simulink model "CompleteModelHiL"  (R2015a)
settings: Solver=ode23  StartTime=0.0  StopTime=20000  RelTol=1e-3
StopFcn:
  | stopfun
values from neighbouring files (symbols this model uses):
  OCV_LUT = block.DialogPrm(1).Data    [AMA_sfunc.m]
undefined symbols (not defined in the file or in its folder): dec_fact, Settings
libraries: dspindex x7, Battery_Unipi x6, dsparch4 x6, simulink x3
settings Model: TunableVars=Bp2,Bp3,Cl,Cs,N,Nbits,OCV_LUT,Qr,R0,Rl,Rs,T,dec_fact,ocv,params_bp,sampletime,soc_bp,soc_init  TunableVarsStorageClass=Auto,Auto,Auto,Auto,Auto,Auto,Auto,Auto,Auto,Auto,Auto,Auto,Auto,Auto,Auto,Auto,Auto,Auto  TunableVarsTypeQualifier=,,,,,,,,,,,,,,,,,  Creator=Rocco  LastModifiedBy=pc2
settings OptimizationCC: InlineParams=on  SimCompilerOptimization=on
settings DebuggingCC: ReadBeforeWriteMsg=DisableAll  WriteAfterWriteMsg=DisableAll  WriteAfterReadMsg=DisableAll  MultiTaskDSMMsg=none
settings ModelReferenceCC: UpdateModelReferenceTargets=IfOutOfDate
settings SFSimCC: SFSimEcho=off

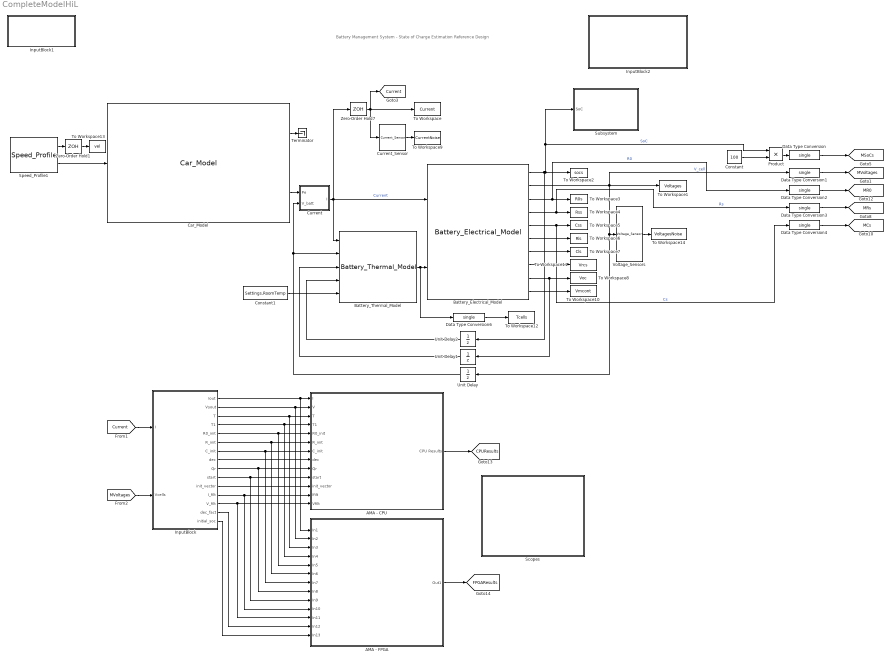
== system CompleteModelHiL ==
  note: Battery Management System - State of Charge Estimation Reference Design
  AMA - CPU : Subsystem
      mask Display: image('cpu.jpg')
  AMA - FPGA : Subsystem
      mask Display: image('max10.jpg')
  Battery_Electrical_Model : Battery_Unipi/Battery_Electrical_Model  N=Settings.N  sampletime=Settings.sampletime  Qbattery=Settings.Q  ocv=Settings.ocv  soc_bp=Settings.soc_bp  params_bp=Settings.params_bp  Ro=Settings.R0lut3d  Rs=Settings.Rslut3d  Cs=Settings.Cslut3d  Rl=Settings.Rllut3d  Cl=Settings.Cllut3d  SoC0=Settings.SoCi  Bp2=Settings.Bp2  Bp3=Settings.Bp3
      link override Cell_Model_therm: R0=Ro
  Battery_Thermal_Model : Battery_Unipi/Battery_Thermal_Model  M=Settings.N/Settings.Strings  Rthca=Settings.ThermRthca  Rthcc=Settings.ThermRthcc  Cth=Settings.ThermCap  Ta=Settings.InitTemp  sampletime=Settings.sampletime
  Car_Model : Battery_Unipi/Car_Model  M=1525  S=2.27  Cx=0.29  alphaR=0.01  roair=1.2  n_wheel=0.7  n_reg=0.5
  Constant : Constant  Value=100
  Constant1 : Constant  Value=Settings.RoomTemp
  Current : Subsystem
  Current_Sensor : Battery_Unipi/Current_Sensor  sampletime=Settings.sampletime  noisevariance=Settings.CurrVar  Nbits=Settings.CurrNbits  FS=Settings.CurrFS  Offset=Settings.CurrOff
  Data Type Conversion{,1..4,6} (6 alike) : DataTypeConversion  OutDataTypeStr=single
  InputBlock : Subsystem
  InputBlock1 : Subsystem
      mask DialogControl altera Prompt: www.altera.com
      mask Display: image('altera-logo-v3.png')
  InputBlock2 : Subsystem
      mask DialogControl altera Prompt: www.unipi.it
      mask Display: image('unipi.jpg')
  Product : Product
  Scopes : Subsystem
      mask Display: image('graph.png')
  Speed_Profile1 : Battery_Unipi/Speed_Profile  selector=Settings.profile
  Subsystem : Subsystem
      mask Display:
      | image('stop.png')
      | port_label('input', 1, 'SoC')
  Terminator : Terminator
  To Workspace : ToWorkspace  VariableName=Current  SaveFormat=Timeseries  SampleTime=-1
  To Workspace1 : ToWorkspace  VariableName=Voltages  SaveFormat=Timeseries  SampleTime=-1
  To Workspace10 : ToWorkspace  VariableName=Vmcont  SaveFormat=Timeseries  SampleTime=-1
      settings: Decimation=10
  To Workspace11 : ToWorkspace  VariableName=Vrcs  SaveFormat=Timeseries  SampleTime=-1
      settings: Decimation=10
  To Workspace12 : ToWorkspace  VariableName=Tcells  SaveFormat=Timeseries  SampleTime=-1
      settings: Decimation=10
  To Workspace13 : ToWorkspace  VariableName=vel  SaveFormat=Timeseries  SampleTime=-1
  To Workspace14 : ToWorkspace  VariableName=VoltagesNoise  SaveFormat=Timeseries  SampleTime=-1
  To Workspace2 : ToWorkspace  VariableName=socs  SaveFormat=Timeseries  SampleTime=-1
  To Workspace3 : ToWorkspace  VariableName=R0s  SaveFormat=Timeseries  SampleTime=-1
      settings: Decimation=10
  To Workspace4 : ToWorkspace  VariableName=Rss  SaveFormat=Timeseries  SampleTime=-1
      settings: Decimation=10
  To Workspace5 : ToWorkspace  VariableName=Css  SaveFormat=Timeseries  SampleTime=-1
      settings: Decimation=10
  To Workspace6 : ToWorkspace  VariableName=Rls  SaveFormat=Timeseries  SampleTime=-1
      settings: Decimation=10
  To Workspace7 : ToWorkspace  VariableName=Cls  SaveFormat=Timeseries  SampleTime=-1
      settings: Decimation=10
  To Workspace8 : ToWorkspace  VariableName=Voc  SaveFormat=Timeseries  SampleTime=-1
      settings: Decimation=10
  To Workspace9 : ToWorkspace  VariableName=CurrentNoise  SaveFormat=Timeseries  SampleTime=-1
  Unit Delay : UnitDelay  InitialCondition=4.16  SampleTime=Settings.sampletime
  Unit Delay1 : UnitDelay  InitialCondition=4.16  SampleTime=Settings.sampletime
  Unit Delay2 : UnitDelay  InitialCondition=Settings.SoCi(1)  SampleTime=Settings.sampletime
  Voltage_Sensors : Battery_Unipi/Voltage_Sensors  sampletime=Settings.sampletime  noisevariance=Settings.VoltVar  Nbits=Settings.VoltNbits  FS=Settings.VoltFS  Offset=Settings.VoltOff
  Zero-Order Hold1 : ZeroOrderHold  SampleTime=Settings.sampletime
  Zero-Order Hold7 : ZeroOrderHold  SampleTime=Settings.sampletime
  tag scope: CPUResults=global, Current=global, FPGAResults=global, MCs=global, MR0=global, MRs=global, MSoCs=global, MVoltages=global
  wires:
  Car_Model/1 -> Terminator/1
  Battery_Electrical_Model/1 -> Unit Delay2/1, Product/1, Subsystem/1(SoC), To Workspace2/1  "SoC"
  Battery_Electrical_Model/2 -> Data Type Conversion1/1, To Workspace1/1, Voltage_Sensors/1, Unit Delay/1  "V_cell"
  Battery_Electrical_Model/5 -> Data Type Conversion4/1, To Workspace5/1  "Cs"
  Battery_Electrical_Model/3 -> Data Type Conversion2/1, To Workspace3/1  "R0"
  Battery_Electrical_Model/4 -> Data Type Conversion3/1, To Workspace4/1  "Rs"
  Battery_Electrical_Model/8 -> To Workspace11/1
  Data Type Conversion6/1 -> To Workspace12/1
  Battery_Electrical_Model/6 -> To Workspace6/1
  Battery_Electrical_Model/7 -> To Workspace7/1
  Car_Model/2 -> Current/1(Pe)
  Zero-Order Hold1/1 -> To Workspace13/1
  Speed_Profile1/1 -> Zero-Order Hold1/1
  Speed_Profile1/2 -> Car_Model/1
  Zero-Order Hold7/1 -> [Current], To Workspace/1, Current_Sensor/1
  Current_Sensor/1 -> To Workspace9/1
  Current/1(I) -> Battery_Electrical_Model/1, Battery_Thermal_Model/1, Zero-Order Hold7/1  "Current"
  Battery_Electrical_Model/10 -> To Workspace10/1
  Battery_Electrical_Model/9 -> Unit Delay1/1, To Workspace8/1
  Voltage_Sensors/1 -> To Workspace14/1
  Battery_Thermal_Model/1 -> Battery_Electrical_Model/2, Data Type Conversion6/1
  Constant1/1 -> Battery_Thermal_Model/5
  Unit Delay/1 -> Battery_Thermal_Model/2, Current/2(V_batt)
  Unit Delay1/1 -> Battery_Thermal_Model/3
  Unit Delay2/1 -> Battery_Thermal_Model/4
  InputBlock/1(Iout) -> AMA - FPGA/1(In1), AMA - CPU/1(I)
  InputBlock/2(Vsout) -> AMA - FPGA/2(In2), AMA - CPU/2(V)
  InputBlock/3(T) -> AMA - FPGA/3(In3), AMA - CPU/3(T)
  InputBlock/4(T1) -> AMA - FPGA/4(In4), AMA - CPU/4(T1)
  InputBlock/6(R_init) -> AMA - FPGA/6(In6), AMA - CPU/6(R_init)
  [Current] -> InputBlock/1(I)
  [MVoltages] -> InputBlock/2(Vcells)
  InputBlock/5("R0_init ") -> AMA - FPGA/5(In5), AMA - CPU/5(R0_init)
  InputBlock/7(C_init) -> AMA - FPGA/7(In7), AMA - CPU/7(C_init)
  InputBlock/8(dec) -> AMA - CPU/8(dec)
  InputBlock/9(Qr) -> AMA - FPGA/8(In8), AMA - CPU/9(Qr)
  InputBlock/10("start ") -> AMA - FPGA/9(In9), AMA - CPU/10(start)
  InputBlock/11(init_vector) -> AMA - CPU/11(init_vector)
  InputBlock/12(I_filt) -> AMA - FPGA/10(In10), AMA - CPU/12(Ifilt)
  InputBlock/13(V_filt) -> AMA - FPGA/11(In11), AMA - CPU/13(Vfilt)
  InputBlock/14(dec_fact) -> AMA - FPGA/12(In12)
  InputBlock/15(initial_soc) -> AMA - FPGA/13(In13)
  AMA - CPU/1(CPU Results) -> [CPUResults]
  AMA - FPGA/1(Out1) -> [FPGAResults]
  Data Type Conversion/1 -> [MSoCs]
  Data Type Conversion1/1 -> [MVoltages]
  Data Type Conversion4/1 -> [MCs]
  Data Type Conversion3/1 -> [MRs]
  Data Type Conversion2/1 -> [MR0]
  Product/1 -> Data Type Conversion/1
  Constant/1 -> Product/2

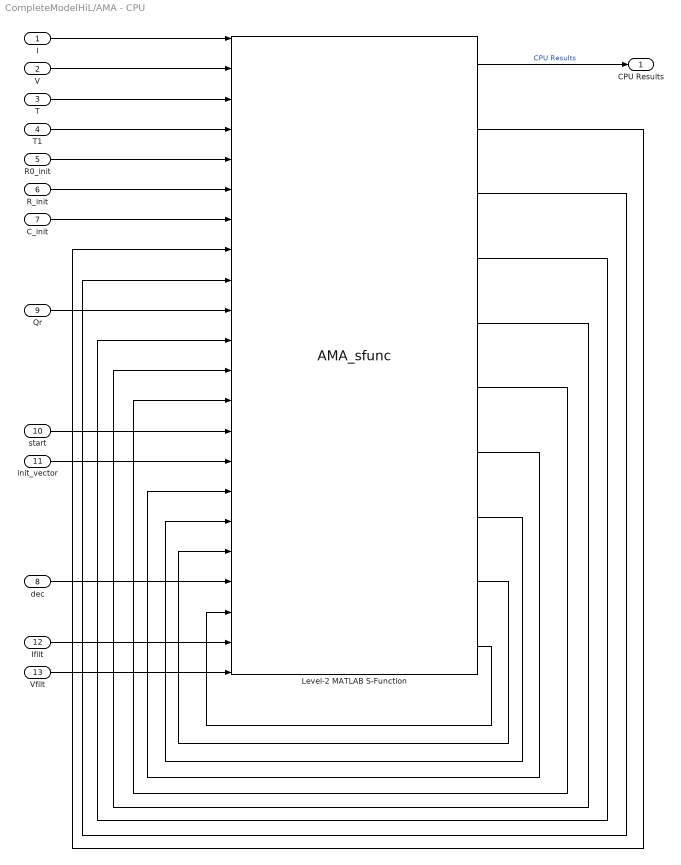
== system CompleteModelHiL/AMA - CPU ==
  I : Inport
  V : Inport  Port=2
  T : Inport  Port=3
  T1 : Inport  Port=4
  R0_init : Inport  Port=5
  R_init : Inport  Port=6
  C_init : Inport  Port=7
  dec : Inport  Port=8
  Qr : Inport  Port=9
  start : Inport  Port=10
  init_vector : Inport  Port=11
  Ifilt : Inport  Port=12
  Vfilt : Inport  Port=13
  Level-2 MATLAB S-Function : M-S-Function  FunctionName=AMA_sfunc  Parameters=single(OCV_LUT)
  CPU Results : Outport
  wires:
  R_init/1 -> Level-2 MATLAB S-Function/6
  V/1 -> Level-2 MATLAB S-Function/2
  dec/1 -> Level-2 MATLAB S-Function/19
  C_init/1 -> Level-2 MATLAB S-Function/7
  I/1 -> Level-2 MATLAB S-Function/1
  T/1 -> Level-2 MATLAB S-Function/3
  T1/1 -> Level-2 MATLAB S-Function/4
  Level-2 MATLAB S-Function/6 -> Level-2 MATLAB S-Function/13
  Level-2 MATLAB S-Function/5 -> Level-2 MATLAB S-Function/12
  Level-2 MATLAB S-Function/2 -> Level-2 MATLAB S-Function/8
  Level-2 MATLAB S-Function/1 -> CPU Results/1  "CPU Results"
  Level-2 MATLAB S-Function/4 -> Level-2 MATLAB S-Function/11
  Level-2 MATLAB S-Function/3 -> Level-2 MATLAB S-Function/9
  Level-2 MATLAB S-Function/9 -> Level-2 MATLAB S-Function/18
  Level-2 MATLAB S-Function/8 -> Level-2 MATLAB S-Function/17
  Level-2 MATLAB S-Function/7 -> Level-2 MATLAB S-Function/16
  Level-2 MATLAB S-Function/10 -> Level-2 MATLAB S-Function/20
  Ifilt/1 -> Level-2 MATLAB S-Function/21
  Vfilt/1 -> Level-2 MATLAB S-Function/22
  R0_init/1 -> Level-2 MATLAB S-Function/5
  Qr/1 -> Level-2 MATLAB S-Function/10
  start/1 -> Level-2 MATLAB S-Function/14
  init_vector/1 -> Level-2 MATLAB S-Function/15

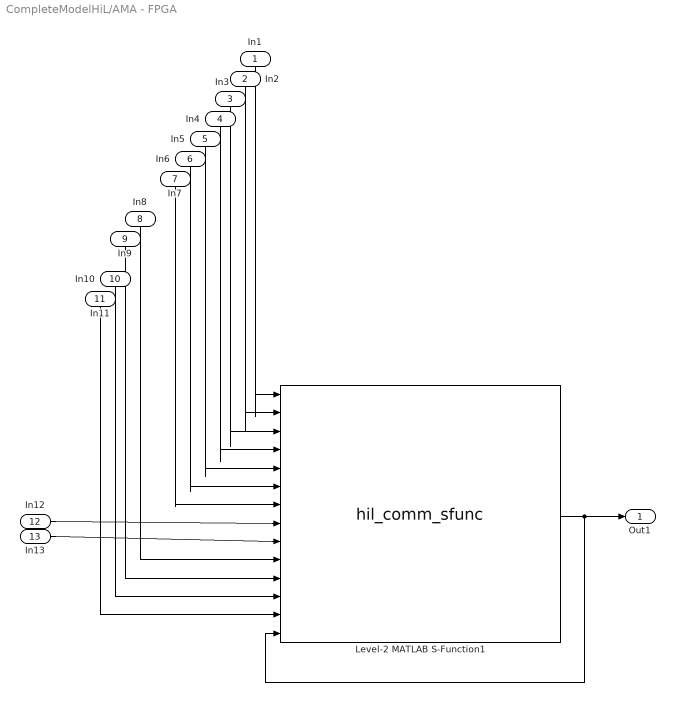
== system CompleteModelHiL/AMA - FPGA ==
  In1 : Inport
  In2 : Inport  Port=2
  In3 : Inport  Port=3
  In4 : Inport  Port=4
  In5 : Inport  Port=5
  In6 : Inport  Port=6
  In7 : Inport  Port=7
  In8 : Inport  Port=8
  In9 : Inport  Port=9
  In10 : Inport  Port=10
  In11 : Inport  Port=11
  In12 : Inport  Port=12
  In13 : Inport  Port=13
  Level-2 MATLAB S-Function1 : M-S-Function  FunctionName=hil_comm_sfunc
  Out1 : Outport
  wires:
  Level-2 MATLAB S-Function1/1 -> Out1/1, Level-2 MATLAB S-Function1/14
  In12/1 -> Level-2 MATLAB S-Function1/8
  In13/1 -> Level-2 MATLAB S-Function1/9
  In3/1 -> Level-2 MATLAB S-Function1/3
  In5/1 -> Level-2 MATLAB S-Function1/5
  In9/1 -> Level-2 MATLAB S-Function1/11
  In6/1 -> Level-2 MATLAB S-Function1/6
  In4/1 -> Level-2 MATLAB S-Function1/4
  In10/1 -> Level-2 MATLAB S-Function1/12
  In11/1 -> Level-2 MATLAB S-Function1/13
  In1/1 -> Level-2 MATLAB S-Function1/1
  In2/1 -> Level-2 MATLAB S-Function1/2
  In7/1 -> Level-2 MATLAB S-Function1/7
  In8/1 -> Level-2 MATLAB S-Function1/10

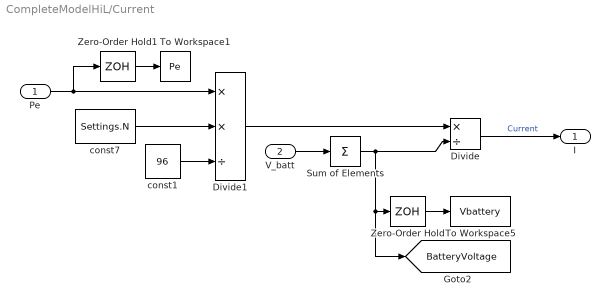
== system CompleteModelHiL/Current ==
  Pe : Inport
  V_batt : Inport  Port=2
  Divide : Product  Inputs=*/
  Divide1 : Product  Inputs=**/
  Sum of Elements : Sum  Inputs=+
  To Workspace1 : ToWorkspace  VariableName=Pe  SaveFormat=Timeseries  SampleTime=-1
      settings: Decimation=10
  To Workspace5 : ToWorkspace  VariableName=Vbattery  SaveFormat=Timeseries  SampleTime=-1
      settings: Decimation=10
  Zero-Order Hold : ZeroOrderHold  SampleTime=Settings.sampletime
  Zero-Order Hold1 : ZeroOrderHold  SampleTime=Settings.sampletime
  const1 : Constant  Value=96  OutDataTypeStr=single  SampleTime=Inf
  const7 : Constant  Value=Settings.N  OutDataTypeStr=single  SampleTime=Inf
  I : Outport
  tag scope: BatteryVoltage=global
  wires:
  Divide1/1 -> Divide/1
  const1/1 -> Divide1/3
  V_batt/1 -> Sum of Elements/1
  Sum of Elements/1 -> Divide/2, [BatteryVoltage], Zero-Order Hold/1
  const7/1 -> Divide1/2
  Pe/1 -> Zero-Order Hold1/1, Divide1/1
  Divide/1 -> I/1  "Current"
  Zero-Order Hold/1 -> To Workspace5/1
  Zero-Order Hold1/1 -> To Workspace1/1

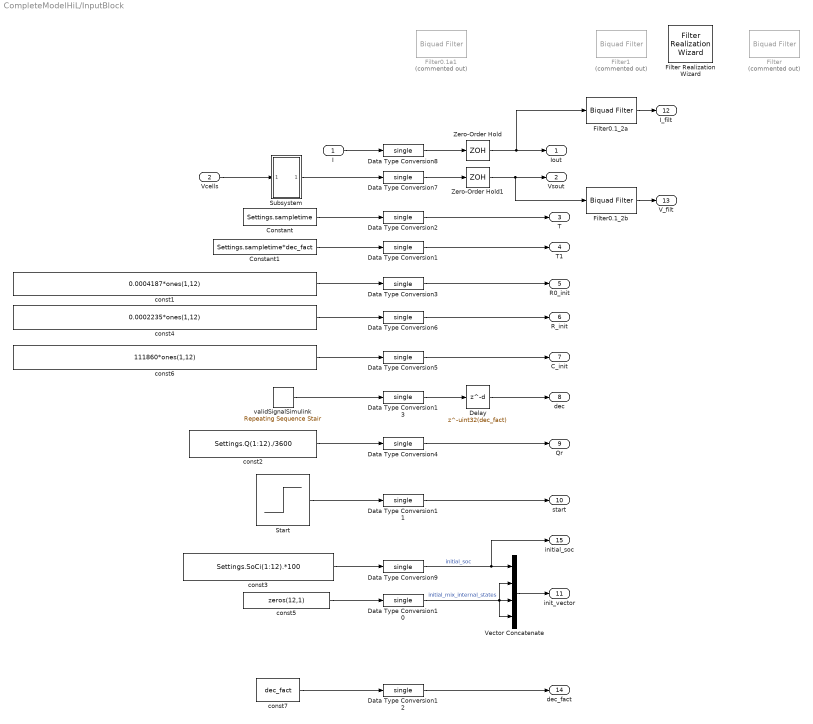
== system CompleteModelHiL/InputBlock ==
  I : Inport
  Vcells : Inport  Port=2
  Constant : Constant  Value=Settings.sampletime  SampleTime=Inf
  Constant1 : Constant  Value=Settings.sampletime*dec_fact  SampleTime=Inf
  Data Type Conversion{1..13} (13 alike) : DataTypeConversion  OutDataTypeStr=single
  Delay : Delay  DelayLength=uint32(dec_fact)  InitialCondition=0  SampleTime=Settings.sampletime
  Filter : dsparch4/Biquad Filter  Tag=BlockMethodSubSystem  Commented=on  IIRFiltStruct=Direct form II  CoeffSource=Specify via dialog  BiQuadCoeffs=[1 -0.37937622398720183 1 1 -1.977761162516769 0.98296154355766985;1 0.057146936114785295 1 1 -1.9491207799698551 0.95293889396365183;1 1.0984661154472131 1 1 -1.9304579283177468 0.93262490079303551;1 1 0 1 -0.96200755126336446 0]  a0Flag=Warning  IC=0  ICnum=0  ICden=0  InputProcessing=Columns as channels (frame based)  denAccumFracLength=30  denProdOutputFracLength=30  secondMemoryFracLength=15  roundingMode=Floor  overflowMode=off  ScaleValues=[0.0019772281687409085;0.0018560239556868123;0.00069936942814560613;0.030829285642533205;1]  optimizeScaleValues=on  ScaleValueMode=Specify via input port (g)  scaleValueFracLength=14  FilterSource=Specify via dialog  FilterObject=Hm_biquad
  Filter Realization Wizard : dsparch4/Filter Realization Wizard
  Filter0.1_2a : dsparch4/Biquad Filter  Tag=BlockMethodSubSystem  IIRFiltStruct=Direct form II  CoeffSource=Specify via dialog  BiQuadCoeffs=[1 1 0 1 -0.99790778897276833 0]  a0Flag=Warning  IC=0  ICnum=0  ICden=0  denAccumFracLength=30  denProdOutputFracLength=30  secondMemoryFracLength=15  roundingMode=Floor  overflowMode=off  ScaleValues=[0.001046105513615904;1]  optimizeScaleValues=on  ScaleValueMode=Specify via input port (g)  scaleValueFracLength=14  FilterSource=Specify via dialog  FilterObject=Hm_biquad
  "Filter0.1_2b " : dsparch4/Biquad Filter  Tag=BlockMethodSubSystem  IIRFiltStruct=Direct form II  CoeffSource=Specify via dialog  BiQuadCoeffs=[1 1 0 1 -0.99790778897276833 0]  a0Flag=Warning  IC=0  ICnum=0  ICden=0  denAccumFracLength=30  denProdOutputFracLength=30  secondMemoryFracLength=15  roundingMode=Floor  overflowMode=off  ScaleValues=[0.001046105513615904;1]  optimizeScaleValues=on  ScaleValueMode=Specify via input port (g)  scaleValueFracLength=14  FilterSource=Specify via dialog  FilterObject=Hm_biquad
  Filter0.1a1 : dsparch4/Biquad Filter  Tag=BlockMethodSubSystem  Commented=on  IIRFiltStruct=Direct form II  CoeffSource=Specify via dialog  BiQuadCoeffs=[1 -1.974309254937566 1 1 -1.9842757746773929 0.98623529999021375;1 -1.9604651825243573 1 1 -1.9593020720948617 0.96094998178536073;1 -1.8754678756966003 1 1 -1.9410248958076679 0.94228507783406268;1 1 0 1 -0.96707816729661034 0]  a0Flag=Warning  IC=0  ICnum=0  ICden=0  denAccumFracLength=30  denProdOutputFracLength=30  secondMemoryFracLength=15  roundingMode=Floor  overflowMode=off  ScaleValues=[0.081260776057318698;0.041682491427062374;0.010119332930712415;0.015450666585834652;1]  optimizeScaleValues=on  ScaleValueMode=Specify via input port (g)  scaleValueFracLength=14  FilterSource=Specify via dialog  FilterObject=Hm_biquad
  Filter1 : dsparch4/Biquad Filter  Tag=BlockMethodSubSystem  Commented=on  IIRFiltStruct=Direct form II  CoeffSource=Specify via dialog  BiQuadCoeffs=[1 -1.7798091534496587 1 1 -1.9420457145983858 0.95939749742566494;1 -1.6698605330873366 1 1 -1.8732930828757175 0.8875398987247719;1 -1.1017802038646665 1 1 -1.8258831781403617 0.83659394313774715;1 1 0 1 -0.90432244987210342 0]  a0Flag=Warning  IC=0  ICnum=0  ICden=0  denAccumFracLength=30  denProdOutputFracLength=30  secondMemoryFracLength=15  roundingMode=Floor  overflowMode=off  ScaleValues=[0.083955978843298612;0.043153931222719252;0.011924436583862363;0.044902783514339607;1]  optimizeScaleValues=on  ScaleValueMode=Specify via input port (g)  scaleValueFracLength=14  FilterSource=Specify via dialog  FilterObject=Hm_biquad
  Start : Step  Time=Settings.sampletime  Before=1  After=0  SampleTime=Settings.sampletime
      mask Display: image('engine_start.jpg')
  Subsystem : Subsystem
  Vector Concatenate : Concatenate  NumInputs=4  Mode=Multidimensional array  ConcatenateDimension=2
  Zero-Order Hold : ZeroOrderHold  SampleTime=Settings.sampletime
  Zero-Order Hold1 : ZeroOrderHold  SampleTime=Settings.sampletime
  const1 : Constant  Value=0.0004187*ones(1,12)  OutDataTypeStr=single  SampleTime=Inf
  const2 : Constant  Value=Settings.Q(1:12)./3600  OutDataTypeStr=single  SampleTime=Inf
  const3 : Constant  Value=Settings.SoCi(1:12).*100  OutDataTypeStr=single  SampleTime=Inf
  const4 : Constant  Value=0.0002235*ones(1,12)  OutDataTypeStr=single  SampleTime=Inf
  const5 : Constant  Value=zeros(12,1)  OutDataTypeStr=single  SampleTime=Inf
  const6 : Constant  Value=111860*ones(1,12)  OutDataTypeStr=single  SampleTime=Inf
  const7 : Constant  Value=dec_fact  OutDataTypeStr=single  SampleTime=Inf
  validSignalSimulink : simulink/Sources/Repeating Sequence Stair  OutValues=[1 zeros(1,dec_fact-1)]  tsamp=Settings.sampletime  OutMin=[]  OutMax=[]  OutDataTypeStr=fixdt('boolean')  OutputDataTypeScalingMode=Specify via dialog  OutDataType=fixdt('boolean')  ConRadixGroup=Best Precision: Vector-wise  OutScaling=[]
  Iout : Outport
  Vsout : Outport  Port=2
  T : Outport  Port=3
  T1 : Outport  Port=4
  "R0_init " : Outport  Port=5
  R_init : Outport  Port=6
  C_init : Outport  Port=7
  dec : Outport  Port=8
  Qr : Outport  Port=9
  "start " : Outport  Port=10
  init_vector : Outport  Port=11
  I_filt : Outport  Port=12
  V_filt : Outport  Port=13
  dec_fact : Outport  Port=14
  initial_soc : Outport  Port=15
  wires:
  const4/1 -> Data Type Conversion6/1
  Data Type Conversion1/1 -> T1/1
  Constant1/1 -> Data Type Conversion1/1
  Data Type Conversion2/1 -> T/1
  Constant/1 -> Data Type Conversion2/1
  Data Type Conversion8/1 -> Zero-Order Hold/1
  Data Type Conversion6/1 -> R_init/1
  I/1 -> Data Type Conversion8/1
  const1/1 -> Data Type Conversion3/1
  Data Type Conversion3/1 -> "R0_init "/1
  const6/1 -> Data Type Conversion5/1
  Data Type Conversion5/1 -> C_init/1
  validSignalSimulink/1 -> Data Type Conversion13/1
  Data Type Conversion13/1 -> Delay/1
  Delay/1 -> dec/1
  const2/1 -> Data Type Conversion4/1
  Data Type Conversion4/1 -> Qr/1
  Start/1 -> Data Type Conversion11/1
  Data Type Conversion11/1 -> "start "/1
  const3/1 -> Data Type Conversion9/1
  const5/1 -> Data Type Conversion10/1
  Data Type Conversion10/1 -> Vector Concatenate/2, Vector Concatenate/4, Vector Concatenate/3  "initial_mix_internal_states"
  Data Type Conversion9/1 -> initial_soc/1, Vector Concatenate/1  "initial_soc"
  Vector Concatenate/1 -> init_vector/1
  Zero-Order Hold/1 -> Filter0.1_2a/1, Iout/1
  Filter0.1_2a/1 -> I_filt/1
  "Filter0.1_2b "/1 -> V_filt/1
  const7/1 -> Data Type Conversion12/1
  Data Type Conversion12/1 -> dec_fact/1
  Vcells/1 -> Subsystem/1(In2)
  Subsystem/1(Out2) -> Data Type Conversion7/1
  Data Type Conversion7/1 -> Zero-Order Hold1/1
  Zero-Order Hold1/1 -> "Filter0.1_2b "/1, Vsout/1

== system CompleteModelHiL/InputBlock1 ==

== system CompleteModelHiL/InputBlock2 ==

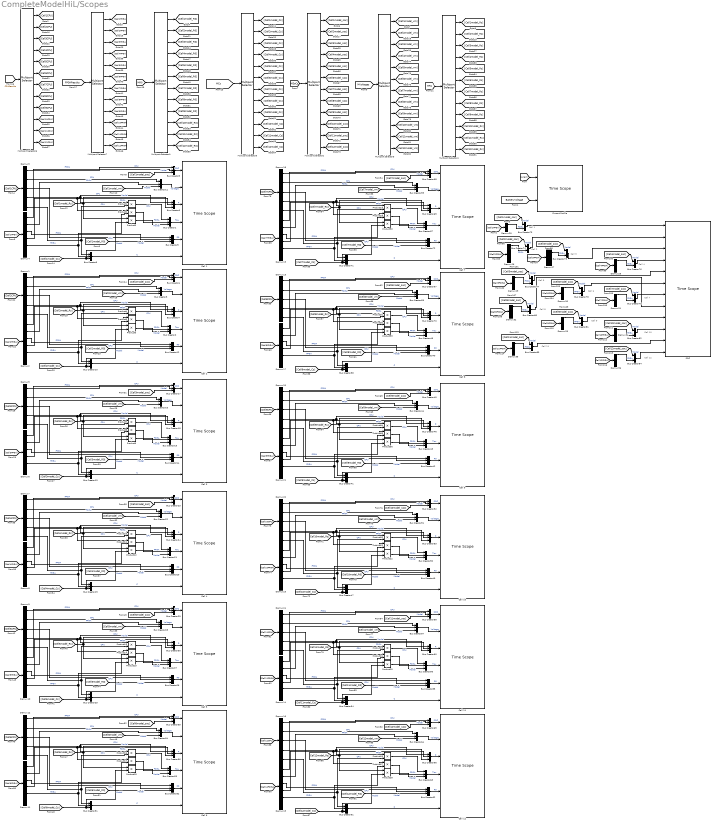
== system CompleteModelHiL/Scopes ==
  note: Cell 1
  note: Cell 2
  note: Cell 3
  note: Cell 4
  note: Cell 5
  note: Cell 6
  note: Cell 7
  note: Cell 8
  note: Cell 9
  note: Cell 10
  note: Cell 11
  note: Cell 12
  Bus Creator{1..72} (72 alike) : BusCreator  Inputs=3
  Bus Creator{73..84} (12 alike) : BusCreator  Inputs=2
  Cell {1..12} (12 alike) : TimeScope  DefaultConfigurationName=spbscopes.TimeScopeBlockCfg  NumInputPorts=6
  Current Profile : TimeScope  DefaultConfigurationName=spbscopes.TimeScopeBlockCfg  NumInputPorts=2
  Demux{1,3,5,7,9,12..13,16,18,20,22,24} (12 alike) : Demux  Outputs=5
  Demux{2,4,6,8,10..11,14..15,17,19,21,23,25..36} (24 alike) : Demux  Outputs=6
  Multiport Selector{1..7} (7 alike) : dspindex/Multiport Selector  rowsOrCols=Rows  idxCellArray={1,2,3,4,5,6,7,8,9,10,11,12 }  idxErrMode=Clip Index
  Product{1..36} (36 alike) : Product
  SOC : TimeScope  DefaultConfigurationName=spbscopes.TimeScopeBlockCfg  NumInputPorts=12
  wires:
  [Cell1model_Cs] -> Product3/2, Bus Creator8/3  "Model"
  [MSoCs] -> Multiport Selector2/1
  [Cell1model_R0] -> Bus Creator9/3  "Model"
  Multiport Selector3/1 -> [Cell1model_vm]
  Multiport Selector5/1 -> [Cell1model_Cs]
  Bus Creator11/1 -> Cell 1/2  "Voltage"
  Demux3/4 -> Bus Creator6/1, Product1/1  "CPU"
  Demux4/1 -> Bus Creator5/2  "FPGA"
  Bus Creator6/1 -> Cell 1/3  "R"
  Demux3/1 -> Bus Creator5/1  "CPU"
  Demux4/2 -> Bus Creator11/2  "FPGA"
  Multiport Selector2/1 -> [Cell1model_soc]
  Bus Creator5/1 -> Cell 1/1  "SOC"
  Product1/1 -> Bus Creator1/1  "CPU"
  Bus Creator8/1 -> Cell 1/6  "C"
  Bus Creator9/1 -> Cell 1/5  "R0"
  Demux3/2 -> Bus Creator11/1  "CPU"
  Multiport Selector5/11 -> [Cell11model_Cs]
  Multiport Selector2/4 -> [Cell4model_soc]
  Multiport Selector2/5 -> [Cell5model_soc]
  Multiport Selector3/8 -> [Cell8model_vm]
  Multiport Selector2/6 -> [Cell6model_soc]
  Product6/1 -> Bus Creator2/3  "Model"
  [Cell2CPU] -> Demux1/1
  Bus Creator4/1 -> Cell 2/1  "SOC"
  Multiport Selector1/3 -> [Cell3model_R0]
  Demux1/4 -> Product4/1, Bus Creator7/1  "CPU"
  Bus Creator3/1 -> Cell 2/2  "Voltage"
  Product4/1 -> Bus Creator2/1  "CPU"
  Multiport Selector3/3 -> [Cell3model_vm]
  Multiport Selector3/9 -> [Cell9model_vm]
  Demux1/2 -> Bus Creator3/1  "CPU"
  [CPUResults] -> Multiport Selector6/1
  [Cell2model_soc] -> Bus Creator4/3  "Model"
  Bus Creator7/1 -> Cell 2/3  "R"
  Demux2/4 -> Bus Creator7/2, Product5/1  "FPGA"
  Demux2/3 -> Bus Creator12/2  "FPGA"
  Demux2/1 -> Bus Creator4/2  "FPGA"
  Demux1/3 -> Bus Creator12/1  "CPU"
  Demux1/5 -> Bus Creator10/1, Product4/2  "CPU"
  [Cell2model_Cs] -> Bus Creator10/3, Product6/2  "Model"
  [Cell2model_vm] -> Bus Creator3/3  "Model"
  Multiport Selector3/6 -> [Cell6model_vm]
  Multiport Selector3/4 -> [Cell4model_vm]
  [Cell2model_Rs] -> Bus Creator7/3, Product6/1  "Model"
  Demux2/5 -> Bus Creator10/2, Product5/2  "FPGA"
  Bus Creator10/1 -> Cell 2/6  "C"
  Product5/1 -> Bus Creator2/2  "FPGA"
  [Cell2model_R0] -> Bus Creator12/3  "Model"
  Multiport Selector7/3 -> [Cell3FPGA]
  Bus Creator2/1 -> Cell 2/4  "Tau"
  Multiport Selector2/3 -> [Cell3model_soc]
  Demux2/2 -> Bus Creator3/2  "FPGA"
  Bus Creator12/1 -> Cell 2/5  "R0"
  Multiport Selector1/7 -> [Cell7model_R0]
  [Cell2FPGA] -> Demux2/1
  Demux1/1 -> Bus Creator4/1  "CPU"
  Multiport Selector6/5 -> [Cell5CPU]
  Multiport Selector2/10 -> [Cell10model_soc]
  Multiport Selector1/11 -> [Cell11model_R0]
  Multiport Selector7/4 -> [Cell4FPGA]
  Multiport Selector3/5 -> [Cell5model_vm]
  Multiport Selector7/9 -> [Cell9FPGA]
  Multiport Selector2/11 -> [Cell11model_soc]
  Multiport Selector1/5 -> [Cell5model_R0]
  Multiport Selector6/2 -> [Cell2CPU]
  Multiport Selector4/5 -> [Cell5model_Rs]
  Multiport Selector7/5 -> [Cell5FPGA]
  Multiport Selector5/7 -> [Cell7model_Cs]
  Multiport Selector4/12 -> [Cell12model_Rs]
  Multiport Selector4/8 -> [Cell8model_Rs]
  Multiport Selector1/4 -> [Cell4model_R0]
  Multiport Selector4/3 -> [Cell3model_Rs]
  Multiport Selector3/2 -> [Cell2model_vm]
  Multiport Selector4/4 -> [Cell4model_Rs]
  Multiport Selector4/9 -> [Cell9model_Rs]
  Multiport Selector2/12 -> [Cell12model_soc]
  Multiport Selector7/10 -> [Cell10FPGA]
  Multiport Selector1/10 -> [Cell10model_R0]
  Multiport Selector2/2 -> [Cell2model_soc]
  Multiport Selector5/9 -> [Cell9model_Cs]
  Multiport Selector2/7 -> [Cell7model_soc]
  Multiport Selector5/2 -> [Cell2model_Cs]
  Multiport Selector3/12 -> [Cell12model_vm]
  Multiport Selector5/3 -> [Cell3model_Cs]
  Multiport Selector7/2 -> [Cell2FPGA]
  Multiport Selector5/5 -> [Cell5model_Cs]
  Multiport Selector1/12 -> [Cell12model_R0]
  Multiport Selector1/6 -> [Cell6model_R0]
  Multiport Selector1/8 -> [Cell8model_R0]
  Multiport Selector6/4 -> [Cell4CPU]
  Multiport Selector7/1 -> [Cell1FPGA]
  Demux4/3 -> Bus Creator9/2  "FPGA"
  Demux3/3 -> Bus Creator9/1  "CPU"
  Demux3/5 -> Product1/2, Bus Creator8/1  "CPU"
  [MCs] -> Multiport Selector5/1
  [Cell1CPU] -> Demux3/1
  [MRs] -> Multiport Selector4/1
  [Cell1FPGA] -> Demux4/1
  Demux4/5 -> Product2/2, Bus Creator8/2  "FPGA"
  Multiport Selector4/1 -> [Cell1model_Rs]
  [Cell1model_Rs] -> Product3/1, Bus Creator6/3  "Model"
  [Cell1model_vm] -> Bus Creator11/3  "Model"
  [MVoltages] -> Multiport Selector3/1
  Demux4/4 -> Product2/1, Bus Creator6/2  "FPGA"
  Multiport Selector6/1 -> [Cell1CPU]
  [MR0] -> Multiport Selector1/1
  [Cell1model_soc] -> Bus Creator5/3  "Model"
  Multiport Selector1/1 -> [Cell1model_R0]
  Demux5/5 -> Product7/2, Bus Creator13/1  "CPU"
  Demux5/4 -> Bus Creator18/1, Product7/1  "CPU"
  [Cell5FPGA] -> Demux10/1
  Product7/1 -> Bus Creator15/1  "CPU"
  Demux7/1 -> Bus Creator23/1  "CPU"
  Demux6/2 -> Bus Creator16/2  "FPGA"
  Demux6/5 -> Product8/2, Bus Creator13/2  "FPGA"
  Bus Creator28/1 -> Cell 5/2  "Voltage"
  Multiport Selector6/10 -> [Cell10CPU]
  Bus Creator13/1 -> Cell 3/6  "C"
  [Cell3model_vm] -> Bus Creator16/3  "Model"
  Demux9/5 -> Product13/2, Bus Creator25/1  "CPU"
  Demux10/4 -> Product14/1, Bus Creator30/2  "FPGA"
  Multiport Selector3/7 -> [Cell7model_vm]
  Demux7/2 -> Bus Creator22/1  "CPU"
  Multiport Selector5/10 -> [Cell10model_Cs]
  Multiport Selector7/11 -> [Cell11FPGA]
  Bus Creator26/1 -> Cell 5/5  "R0"
  Bus Creator15/1 -> Cell 3/4  "Tau"
  Multiport Selector1/9 -> [Cell9model_R0]
  Demux8/3 -> Bus Creator20/2  "FPGA"
  Demux10/3 -> Bus Creator26/2  "FPGA"
  Product15/1 -> Bus Creator27/3  "Model"
  Product10/1 -> Bus Creator21/1  "CPU"
  Product11/1 -> Bus Creator21/2  "FPGA"
  Product13/1 -> Bus Creator27/1  "CPU"
  Demux6/4 -> Product8/1, Bus Creator18/2  "FPGA"
  Multiport Selector4/10 -> [Cell10model_Rs]
  Demux8/4 -> Bus Creator24/2, Product11/1  "FPGA"
  Multiport Selector6/7 -> [Cell7CPU]
  [Cell5model_Cs] -> Product15/2, Bus Creator25/3  "Model"
  Demux8/1 -> Bus Creator23/2  "FPGA"
  [Cell5model_Rs] -> Product15/1, Bus Creator30/3  "Model"
  Demux10/1 -> Bus Creator29/2  "FPGA"
  Multiport Selector6/3 -> [Cell3CPU]
  [Cell3CPU] -> Demux5/1
  Multiport Selector4/2 -> [Cell2model_Rs]
  Multiport Selector3/10 -> [Cell10model_vm]
  Multiport Selector5/6 -> [Cell6model_Cs]
  [Cell5model_vm] -> Bus Creator28/3  "Model"
  Bus Creator27/1 -> Cell 5/4  "Tau"
  Product12/1 -> Bus Creator21/3  "Model"
  Bus Creator24/1 -> Cell 4/3  "R"
  Demux6/3 -> Bus Creator14/2  "FPGA"
  Multiport Selector7/7 -> [Cell7FPGA]
  Multiport Selector5/12 -> [Cell12model_Cs]
  [Cell4model_Cs] -> Bus Creator19/3, Product12/2  "Model"
  [Cell5CPU] -> Demux9/1
  [Cell3model_R0] -> Bus Creator14/3  "Model"
  Demux9/3 -> Bus Creator26/1  "CPU"
  [Cell4model_vm] -> Bus Creator22/3  "Model"
  Multiport Selector4/7 -> [Cell7model_Rs]
  Multiport Selector7/6 -> [Cell6FPGA]
  [Cell3FPGA] -> Demux6/1
  Multiport Selector6/8 -> [Cell8CPU]
  Demux5/3 -> Bus Creator14/1  "CPU"
  Bus Creator14/1 -> Cell 3/5  "R0"
  Bus Creator17/1 -> Cell 3/1  "SOC"
  [Cell3model_Rs] -> Product9/1, Bus Creator18/3  "Model"
  [Cell3model_Cs] -> Product9/2, Bus Creator13/3  "Model"
  Demux5/1 -> Bus Creator17/1  "CPU"
  Multiport Selector4/11 -> [Cell11model_Rs]
  Bus Creator21/1 -> Cell 4/4  "Tau"
  Demux9/4 -> Bus Creator30/1, Product13/1  "CPU"
  Bus Creator18/1 -> Cell 3/3  "R"
  Multiport Selector4/6 -> [Cell6model_Rs]
  Bus Creator19/1 -> Cell 4/6  "C"
  Demux9/2 -> Bus Creator28/1  "CPU"
  Multiport Selector5/4 -> [Cell4model_Cs]
  Multiport Selector6/11 -> [Cell11CPU]
  Multiport Selector7/12 -> [Cell12FPGA]
  Demux7/4 -> Product10/1, Bus Creator24/1  "CPU"
  Demux6/1 -> Bus Creator17/2  "FPGA"
  [FPGAResults] -> Multiport Selector7/1
  Multiport Selector2/9 -> [Cell9model_soc]
  Multiport Selector1/2 -> [Cell2model_R0]
  Multiport Selector7/8 -> [Cell8FPGA]
  Bus Creator16/1 -> Cell 3/2  "Voltage"
  Product8/1 -> Bus Creator15/2  "FPGA"
  [Cell3model_soc] -> Bus Creator17/3  "Model"
  Multiport Selector6/12 -> [Cell12CPU]
  Multiport Selector6/6 -> [Cell6CPU]
  Demux8/5 -> Bus Creator19/2, Product11/2  "FPGA"
  Product14/1 -> Bus Creator27/2  "FPGA"
  Demux7/5 -> Bus Creator19/1, Product10/2  "CPU"
  Bus Creator20/1 -> Cell 4/5  "R0"
  [Cell4model_Rs] -> Bus Creator24/3, Product12/1  "Model"
  [Cell5model_soc] -> Bus Creator29/3  "Model"
  Demux10/2 -> Bus Creator28/2  "FPGA"
  Bus Creator29/1 -> Cell 5/1  "SOC"
  [Cell5model_R0] -> Bus Creator26/3  "Model"
  [Cell4model_soc] -> Bus Creator23/3  "Model"
  Multiport Selector3/11 -> [Cell11model_vm]
  Demux10/5 -> Product14/2, Bus Creator25/2  "FPGA"
  Demux5/2 -> Bus Creator16/1  "CPU"
  Product9/1 -> Bus Creator15/3  "Model"
  Bus Creator25/1 -> Cell 5/6  "C"
  [Cell4FPGA] -> Demux8/1
  Multiport Selector5/8 -> [Cell8model_Cs]
  Bus Creator22/1 -> Cell 4/2  "Voltage"
  [Cell4model_R0] -> Bus Creator20/3  "Model"
  Demux7/3 -> Bus Creator20/1  "CPU"
  Multiport Selector6/9 -> [Cell9CPU]
  [Cell4CPU] -> Demux7/1
  Bus Creator30/1 -> Cell 5/3  "R"
  Demux9/1 -> Bus Creator29/1  "CPU"
  Multiport Selector2/8 -> [Cell8model_soc]
  Demux8/2 -> Bus Creator22/2  "FPGA"
  Bus Creator23/1 -> Cell 4/1  "SOC"
  Product21/1 -> Bus Creator50/2  "FPGA"
  Bus Creator57/1 -> Cell 11/2  "Voltage"
  Bus Creator48/1 -> Cell 8/4  "Tau"
  Demux11/4 -> Bus Creator36/2, Product17/1  "FPGA"
  Demux16/2 -> Bus Creator64/1  "CPU"
  [Cell10CPU] -> Demux22/1
  Bus Creator42/1 -> Cell 9/5  "R0"
  Demux14/2 -> Bus Creator57/2  "FPGA"
  Demux19/3 -> Bus Creator72/2  "FPGA"
  [Cell12FPGA] -> Demux15/1
  [Cell6model_soc] -> Bus Creator35/3  "Model"
  Demux21/2 -> Bus Creator44/2  "FPGA"
  [Cell12model_vm] -> Bus Creator64/3  "Model"
  [Cell6model_Cs] -> Bus Creator31/3, Product18/2  "Model"
  Bus Creator69/1 -> Cell 7/3  "R"
  [Cell7model_Rs] -> Bus Creator69/3, Product30/1  "Model"
  Bus Creator43/1 -> Cell 9/4  "Tau"
  Bus Creator58/1 -> Cell 11/1  "SOC"
  Product26/1 -> Bus Creator63/1  "CPU"
  [Cell11model_R0] -> Bus Creator55/3  "Model"
  Product28/1 -> Bus Creator63/3  "Model"
  Product19/1 -> Bus Creator37/1  "CPU"
  Product33/1 -> Bus Creator48/3  "Model"
  Demux11/2 -> Bus Creator34/2  "FPGA"
  Demux24/4 -> Product23/1, Bus Creator60/1  "CPU"
  Demux14/3 -> Bus Creator55/2  "FPGA"
  [Cell12model_soc] -> Bus Creator65/3  "Model"
  Demux16/5 -> Product26/2, Bus Creator61/1  "CPU"
  [Cell11model_Rs] -> Bus Creator60/3, Product25/1  "Model"
  Product25/1 -> Bus Creator56/3  "Model"
  [Cell10model_R0] -> Bus Creator49/3  "Model"
  Bus Creator31/1 -> Cell 6/6  "C"
  Bus Creator49/1 -> Cell 10/5  "R0"
  Demux13/5 -> Product31/2, Bus Creator38/1  "CPU"
  Demux17/1 -> Bus Creator67/2  "FPGA"
  Bus Creator46/1 -> Cell 9/3  "R"
  Demux16/1 -> Bus Creator65/1  "CPU"
  Demux19/4 -> Bus Creator69/2, Product29/1  "FPGA"
  Demux17/4 -> Product32/1, Bus Creator70/2  "FPGA"
  Bus Creator61/1 -> Cell 12/6  "C"
  [Cell7model_soc] -> Bus Creator68/3  "Model"
  [Cell7FPGA] -> Demux19/1
  [Cell8model_soc] -> Bus Creator67/3  "Model"
  Demux13/2 -> Bus Creator59/1  "CPU"
  Demux15/5 -> Product27/2, Bus Creator61/2  "FPGA"
  Bus Creator47/1 -> Cell 10/6  "C"
  Bus Creator33/1 -> Cell 6/4  "Tau"
  Product36/1 -> Bus Creator43/3  "Model"
  [Cell7model_vm] -> Bus Creator39/3  "Model"
  Product32/1 -> Bus Creator48/2  "FPGA"
  Demux23/1 -> Bus Creator52/2  "FPGA"
  Bus Creator37/1 -> Cell 7/4  "Tau"
  Bus Creator50/1 -> Cell 10/4  "Tau"
  Demux19/2 -> Bus Creator39/2  "FPGA"
  Bus Creator34/1 -> Cell 6/2  "Voltage"
  Bus Creator72/1 -> Cell 7/5  "R0"
  Bus Creator40/1 -> Cell 8/5  "R0"
  Bus Creator41/1 -> Cell 9/6  "C"
  Demux16/4 -> Bus Creator66/1, Product26/1  "CPU"
  Demux20/4 -> Product34/1, Bus Creator46/1  "CPU"
  Demux13/1 -> Bus Creator67/1  "CPU"
  Bus Creator65/1 -> Cell 12/1  "SOC"
  Product27/1 -> Bus Creator63/2  "FPGA"
  [Cell8model_vm] -> Bus Creator59/3  "Model"
  [Cell11model_vm] -> Bus Creator57/3  "Model"
  Demux14/5 -> Bus Creator54/2, Product24/2  "FPGA"
  Demux12/1 -> Bus Creator35/1  "CPU"
  Product22/1 -> Bus Creator50/3  "Model"
  Bus Creator39/1 -> Cell 7/2  "Voltage"
  Bus Creator67/1 -> Cell 8/1  "SOC"
  [Cell12model_Cs] -> Product28/2, Bus Creator61/3  "Model"
  Bus Creator64/1 -> Cell 12/2  "Voltage"
  Demux24/2 -> Bus Creator57/1  "CPU"
  [Cell7model_R0] -> Bus Creator72/3  "Model"
  Demux23/3 -> Bus Creator49/2  "FPGA"
  Bus Creator53/1 -> Cell 10/3  "R"
  Bus Creator56/1 -> Cell 11/4  "Tau"
  Demux22/3 -> Bus Creator49/1  "CPU"
  [Cell11CPU] -> Demux24/1
  Demux14/4 -> Bus Creator60/2, Product24/1  "FPGA"
  Bus Creator55/1 -> Cell 11/5  "R0"
  [Cell11model_soc] -> Bus Creator58/3  "Model"
  Demux18/2 -> Bus Creator39/1  "CPU"
  Bus Creator54/1 -> Cell 11/6  "C"
  Bus Creator66/1 -> Cell 12/3  "R"
  Bus Creator51/1 -> Cell 10/2  "Voltage"
  [Cell10model_Rs] -> Product22/1, Bus Creator53/3  "Model"
  Demux17/2 -> Bus Creator59/2  "FPGA"
  Bus Creator68/1 -> Cell 7/1  "SOC"
  Demux21/4 -> Bus Creator46/2, Product35/1  "FPGA"
  Demux24/1 -> Bus Creator58/1  "CPU"
  Demux19/5 -> Bus Creator71/2, Product29/2  "FPGA"
  [Cell9CPU] -> Demux20/1
  [Cell9FPGA] -> Demux21/1
  Bus Creator59/1 -> Cell 8/2  "Voltage"
  [Cell8model_R0] -> Bus Creator40/3  "Model"
  [Cell12model_Rs] -> Product28/1, Bus Creator66/3  "Model"
  Demux16/3 -> Bus Creator62/1  "CPU"
  [Cell7CPU] -> Demux18/1
  [Cell10FPGA] -> Demux23/1
  Demux15/2 -> Bus Creator64/2  "FPGA"
  Bus Creator63/1 -> Cell 12/4  "Tau"
  Product30/1 -> Bus Creator37/3  "Model"
  Demux11/5 -> Bus Creator31/2, Product17/2  "FPGA"
  Demux20/1 -> Bus Creator45/1  "CPU"
  Demux17/5 -> Product32/2, Bus Creator38/2  "FPGA"
  Demux12/2 -> Bus Creator34/1  "CPU"
  Bus Creator44/1 -> Cell 9/2  "Voltage"
  Product16/1 -> Bus Creator33/1  "CPU"
  [Cell6model_R0] -> Bus Creator32/3  "Model"
  Demux24/3 -> Bus Creator55/1  "CPU"
  Demux24/5 -> Bus Creator54/1, Product23/2  "CPU"
  Product18/1 -> Bus Creator33/3  "Model"
  Bus Creator60/1 -> Cell 11/3  "R"
  Product24/1 -> Bus Creator56/2  "FPGA"
  [Cell11model_Cs] -> Bus Creator54/3, Product25/2  "Model"
  Demux23/4 -> Product21/1, Bus Creator53/2  "FPGA"
  [Cell9model_soc] -> Bus Creator45/3  "Model"
  Demux20/5 -> Bus Creator41/1, Product34/2  "CPU"
  Product34/1 -> Bus Creator43/1  "CPU"
  Bus Creator45/1 -> Cell 9/1  "SOC"
  Demux18/4 -> Product19/1, Bus Creator69/1  "CPU"
  Demux21/3 -> Bus Creator42/2  "FPGA"
  Demux21/1 -> Bus Creator45/2  "FPGA"
  Demux23/5 -> Product21/2, Bus Creator47/2  "FPGA"
  Demux15/3 -> Bus Creator62/2  "FPGA"
  Product35/1 -> Bus Creator43/2  "FPGA"
  [Cell6FPGA] -> Demux11/1
  [Cell7model_Cs] -> Bus Creator71/3, Product30/2  "Model"
  [Cell9model_Rs] -> Bus Creator46/3, Product36/1  "Model"
  [Cell6model_vm] -> Bus Creator34/3  "Model"
  [Cell8model_Cs] -> Product33/2, Bus Creator38/3  "Model"
  Demux20/3 -> Bus Creator42/1  "CPU"
  Demux20/2 -> Bus Creator44/1  "CPU"
  Demux18/1 -> Bus Creator68/1  "CPU"
  [Cell8CPU] -> Demux13/1
  Demux15/1 -> Bus Creator65/2  "FPGA"
  Demux19/1 -> Bus Creator68/2  "FPGA"
  Bus Creator71/1 -> Cell 7/6  "C"
  [Cell10model_Cs] -> Product22/2, Bus Creator47/3  "Model"
  [Cell10model_soc] -> Bus Creator52/3  "Model"
  Product23/1 -> Bus Creator56/1  "CPU"
  [Cell6model_Rs] -> Bus Creator36/3, Product18/1  "Model"
  Product17/1 -> Bus Creator33/2  "FPGA"
  [Cell9model_R0] -> Bus Creator42/3  "Model"
  [Cell12CPU] -> Demux16/1
  Demux12/4 -> Product16/1, Bus Creator36/1  "CPU"
  Product29/1 -> Bus Creator37/2  "FPGA"
  Bus Creator62/1 -> Cell 12/5  "R0"
  Demux22/1 -> Bus Creator52/1  "CPU"
  [Cell8FPGA] -> Demux17/1
  Demux12/5 -> Bus Creator31/1, Product16/2  "CPU"
  [Cell9model_vm] -> Bus Creator44/3  "Model"
  [Cell12model_R0] -> Bus Creator62/3  "Model"
  Demux22/2 -> Bus Creator51/1  "CPU"
  Demux11/3 -> Bus Creator32/2  "FPGA"
  Demux13/4 -> Bus Creator70/1, Product31/1  "CPU"
  Product20/1 -> Bus Creator50/1  "CPU"
  Demux11/1 -> Bus Creator35/2  "FPGA"
  [Cell6CPU] -> Demux12/1
  [Cell11FPGA] -> Demux14/1
  Demux21/5 -> Bus Creator41/2, Product35/2  "FPGA"
  Demux18/5 -> Bus Creator71/1, Product19/2  "CPU"
  [Cell9model_Cs] -> Bus Creator41/3, Product36/2  "Model"
  Product31/1 -> Bus Creator48/1  "CPU"
  Bus Creator32/1 -> Cell 6/5  "R0"
  Demux18/3 -> Bus Creator72/1  "CPU"
  Demux12/3 -> Bus Creator32/1  "CPU"
  Bus Creator35/1 -> Cell 6/1  "SOC"
  Bus Creator52/1 -> Cell 10/1  "SOC"
  [Cell8model_Rs] -> Product33/1, Bus Creator70/3  "Model"
  Demux17/3 -> Bus Creator40/2  "FPGA"
  Bus Creator36/1 -> Cell 6/3  "R"
  Demux14/1 -> Bus Creator58/2  "FPGA"
  Demux22/5 -> Product20/2, Bus Creator47/1  "CPU"
  Bus Creator38/1 -> Cell 8/6  "C"
  Demux15/4 -> Product27/1, Bus Creator66/2  "FPGA"
  [Cell10model_vm] -> Bus Creator51/3  "Model"
  Bus Creator70/1 -> Cell 8/3  "R"
  Demux23/2 -> Bus Creator51/2  "FPGA"
  Demux13/3 -> Bus Creator40/1  "CPU"
  Demux22/4 -> Bus Creator53/1, Product20/1  "CPU"
  Bus Creator1/1 -> Cell 1/4  "Tau"
  Product3/1 -> Bus Creator1/3  "Model"
  Product2/1 -> Bus Creator1/2  "FPGA"
  [Current] -> Current Profile/1
  [BatteryVoltage] -> Current Profile/2
  Bus Creator73/1 -> SOC/1
  Demux25/1 -> Bus Creator73/2  "FPGA"
  [Cell1FPGA] -> Demux25/1
  [Cell1model_soc] -> Bus Creator73/1  "Model"
  Bus Creator74/1 -> SOC/2
  Demux26/1 -> Bus Creator74/2  "FPGA"
  [Cell2FPGA] -> Demux26/1
  [Cell2model_soc] -> Bus Creator74/1  "Model"
  Bus Creator75/1 -> SOC/3
  Demux27/1 -> Bus Creator75/2  "FPGA"
  [Cell3FPGA] -> Demux27/1
  [Cell3model_soc] -> Bus Creator75/1  "Model"
  Demux28/1 -> Bus Creator76/2  "FPGA"
  [Cell4FPGA] -> Demux28/1
  [Cell4model_soc] -> Bus Creator76/1  "Model"
  Bus Creator76/1 -> SOC/4
  Demux29/1 -> Bus Creator77/2  "FPGA"
  [Cell5FPGA] -> Demux29/1
  [Cell5model_soc] -> Bus Creator77/1  "Model"
  Bus Creator77/1 -> SOC/5
  Demux30/1 -> Bus Creator78/2  "FPGA"
  [Cell6FPGA] -> Demux30/1
  [Cell6model_soc] -> Bus Creator78/1  "Model"
  Bus Creator78/1 -> SOC/6
  Demux31/1 -> Bus Creator79/2  "FPGA"
  [Cell7FPGA] -> Demux31/1
  [Cell7model_soc] -> Bus Creator79/1  "Model"
  Bus Creator79/1 -> SOC/7
  Demux32/1 -> Bus Creator80/2  "FPGA"
  [Cell8FPGA] -> Demux32/1
  [Cell8model_soc] -> Bus Creator80/1  "Model"
  Bus Creator80/1 -> SOC/8
  Demux33/1 -> Bus Creator81/2  "FPGA"
  [Cell9FPGA] -> Demux33/1
  [Cell9model_soc] -> Bus Creator81/1  "Model"
  Bus Creator81/1 -> SOC/9
  Demux34/1 -> Bus Creator82/2  "FPGA"
  [Cell10FPGA] -> Demux34/1
  [Cell10model_soc] -> Bus Creator82/1  "Model"
  Bus Creator82/1 -> SOC/10
  Demux35/1 -> Bus Creator83/2  "FPGA"
  [Cell11FPGA] -> Demux35/1
  [Cell11model_soc] -> Bus Creator83/1  "Model"
  Bus Creator83/1 -> SOC/11
  Demux36/1 -> Bus Creator84/2  "FPGA"
  [Cell12FPGA] -> Demux36/1
  [Cell12model_soc] -> Bus Creator84/1  "Model"
  Bus Creator84/1 -> SOC/12

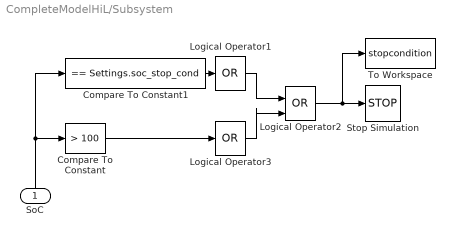
== system CompleteModelHiL/Subsystem ==
  SoC : Inport
  Compare To Constant : simulink/Logic and Bit Operations/Compare To Constant  relop=>  const=100  OutDataTypeStr=boolean
  Compare To Constant1 : simulink/Logic and Bit Operations/Compare To Constant  relop===  const=Settings.soc_stop_cond  OutDataTypeStr=boolean  ZeroCross=off
  Logical Operator1 : Logic  Operator=OR  Inputs=1  IconShape=distinctive  AllPortsSameDT=off  OutDataTypeStr=boolean
  Logical Operator2 : Logic  Operator=OR  IconShape=distinctive  AllPortsSameDT=off  OutDataTypeStr=boolean
  Logical Operator3 : Logic  Operator=OR  Inputs=1  IconShape=distinctive  AllPortsSameDT=off  OutDataTypeStr=boolean
  Stop Simulation : Stop
  To Workspace : ToWorkspace  VariableName=stopcondition  SaveFormat=Timeseries  SampleTime=-1
  wires:
  Compare To Constant/1 -> Logical Operator3/1
  Compare To Constant1/1 -> Logical Operator1/1
  SoC/1 -> Compare To Constant/1, Compare To Constant1/1
  Logical Operator2/1 -> To Workspace/1, Stop Simulation/1
  Logical Operator3/1 -> Logical Operator2/2
  Logical Operator1/1 -> Logical Operator2/1

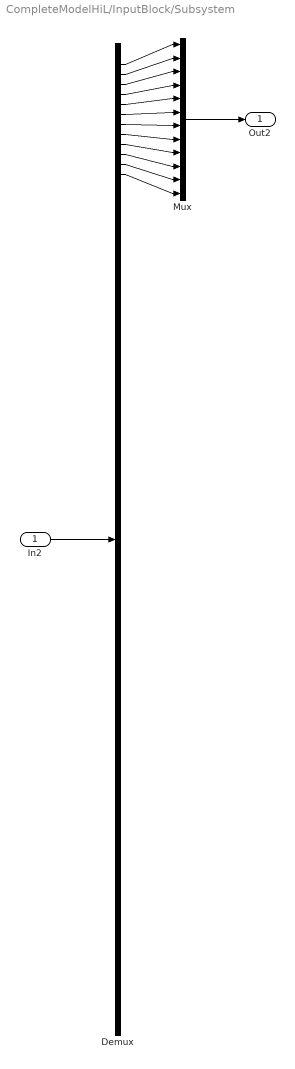
== system CompleteModelHiL/InputBlock/Subsystem ==
  In2 : Inport
  Demux : Demux  Outputs=96
  Mux : Mux  Inputs=12
  Out2 : Outport
  wires:
  Mux/1 -> Out2/1
  In2/1 -> Demux/1
  Demux/1 -> Mux/1
  Demux/2 -> Mux/2
  Demux/3 -> Mux/3
  Demux/4 -> Mux/4
  Demux/5 -> Mux/5
  Demux/6 -> Mux/6
  Demux/7 -> Mux/7
  Demux/8 -> Mux/8
  Demux/9 -> Mux/9
  Demux/10 -> Mux/10
  Demux/11 -> Mux/11
  Demux/12 -> Mux/12
